simulink model "covid"  (R2018b)
settings: Solver=VariableStepAuto  StartTime=0.0  StopTime=10.0  RelTol=1e-3
libraries: fuzblock x1
settings Model: Creator=ARTA  LastModifiedBy=ARTA

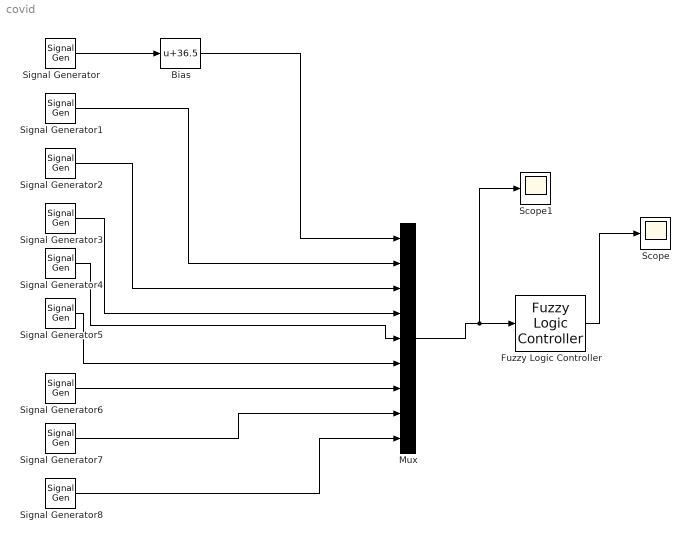
== system covid ==
  Bias : Bias  Bias=36.5
  Fuzzy Logic Controller : fuzblock/Fuzzy Logic  Controller  FIS=covid  OutputSampleNumber=101  DataType=double  FuzzifiedInputs=off  RuleFiringStrengths=off  RuleOutputs=off  AggregatedOutputs=off  SimulateUsing=Interpreted execution  OutOfRangeInputValueMessage=warning  NoRuleFiredMessage=warning  EmptyOutputFuzzySetMessage=warning
  Mux : Mux  Inputs=9
  Scope : Scope
  Scope1 : Scope
  Signal Generator : SignalGenerator  WaveForm=random  Amplitude=5.5  Frequency=0.1  Units=rad/sec
  Signal Generator{1..8} (8 alike) : SignalGenerator  WaveForm=random  Amplitude=5  Frequency=0.1  Units=rad/sec
  wires:
  Fuzzy Logic Controller/1 -> Scope/1
  Signal Generator/1 -> Bias/1
  Mux/1 -> Scope1/1, Fuzzy Logic Controller/1
  Bias/1 -> Mux/1
  Signal Generator1/1 -> Mux/2
  Signal Generator2/1 -> Mux/3
  Signal Generator3/1 -> Mux/4
  Signal Generator4/1 -> Mux/5
  Signal Generator5/1 -> Mux/6
  Signal Generator6/1 -> Mux/7
  Signal Generator7/1 -> Mux/8
  Signal Generator8/1 -> Mux/9
